simulink model "p1"  (R2021a)
settings: Solver=FixedStepAuto  StartTime=0.0  StopTime=10.0  RelTol=1e-3
settings Model: EnablePacing=on  PacingRate=0.100000  Creator=Abbas  LastModifiedBy=Abbas

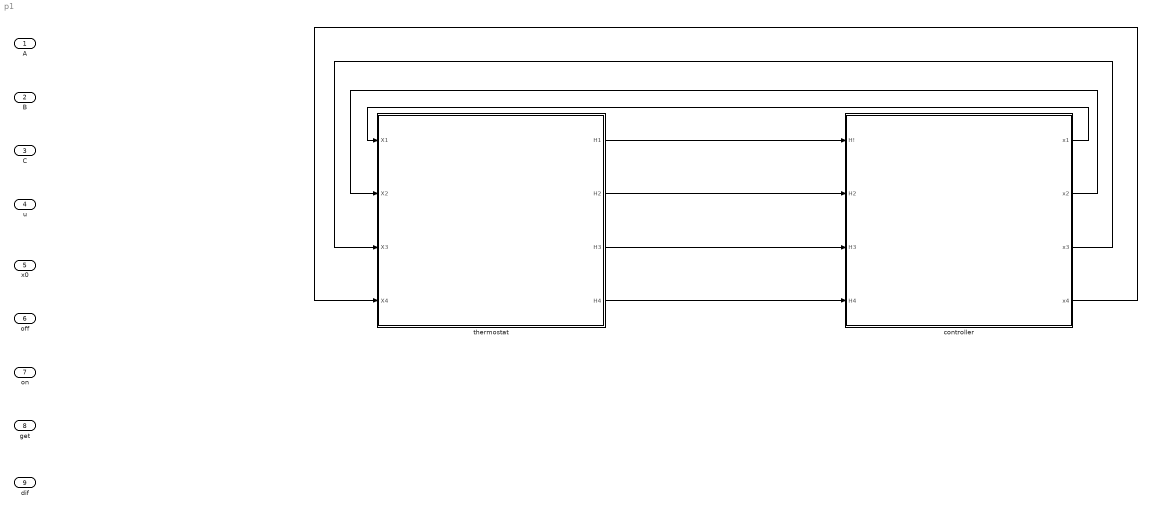
== system p1 ==
  A : Inport
  B : Inport  Port=2
  C : Inport  Port=3
  u : Inport  Port=4
  x0 : Inport  Port=5
  off : Inport  Port=6
  on : Inport  Port=7
  get : Inport  Port=8
  dif : Inport  Port=9
  controller : Subsystem
  thermostat : Subsystem
  wires:
  controller/1(x1) -> thermostat/1(X1)
  thermostat/1(H1) -> controller/1(H!)
  thermostat/2(H2) -> controller/2(H2)
  thermostat/3(H3) -> controller/3(H3)
  thermostat/4(H4) -> controller/4(H4)
  controller/2(x2) -> thermostat/2(X2)
  controller/3(x3) -> thermostat/3(X3)
  controller/4(x4) -> thermostat/4(X4)

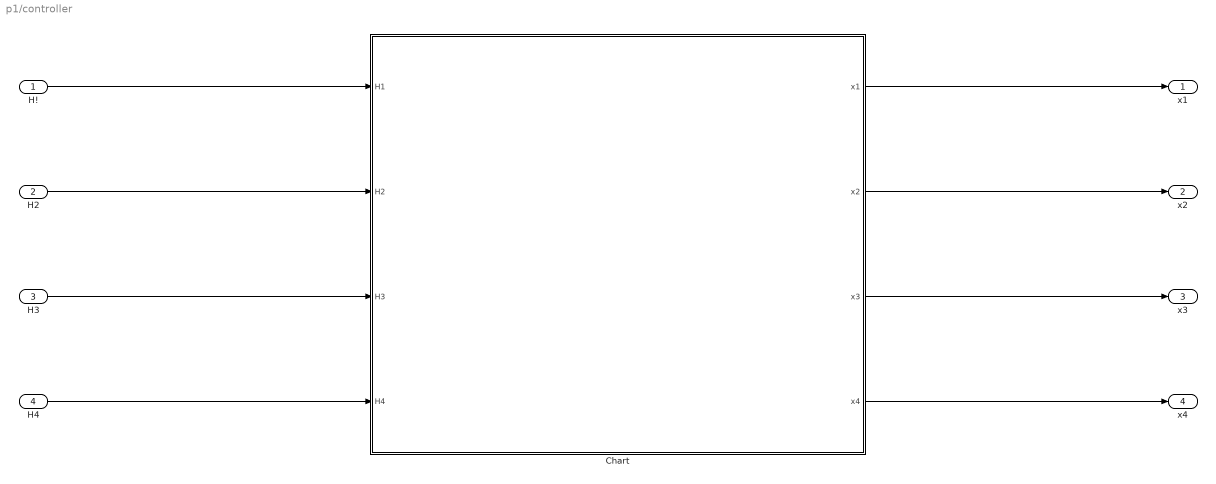
== system p1/controller ==
  H! : Inport
  H2 : Inport  Port=2
  H3 : Inport  Port=3
  H4 : Inport  Port=4
  Chart : Stateflow chart  TreatAsAtomicUnit=on
  x1 : Outport
  x2 : Outport  Port=2
  x3 : Outport  Port=3
  x4 : Outport  Port=4
  wires:
  Chart/1(x1) -> x1/1
  Chart/2(x2) -> x2/1
  Chart/3(x3) -> x3/1
  Chart/4(x4) -> x4/1
  H!/1 -> Chart/1(H1)
  H2/1 -> Chart/2(H2)
  H3/1 -> Chart/3(H3)
  H4/1 -> Chart/4(H4)

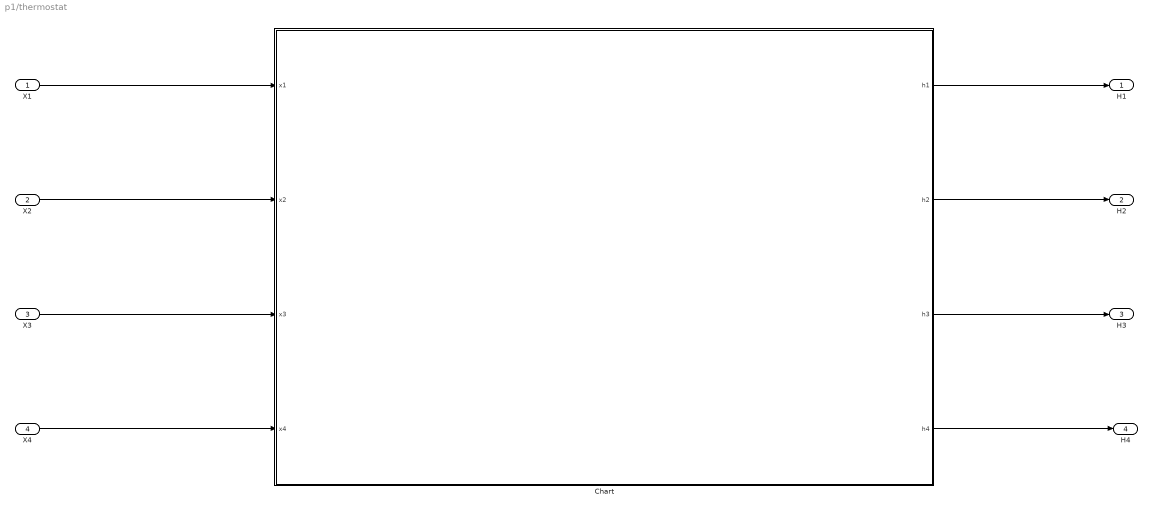
== system p1/thermostat ==
  X1 : Inport
  X2 : Inport  Port=2
  X3 : Inport  Port=3
  X4 : Inport  Port=4
  Chart : Stateflow chart  TreatAsAtomicUnit=on
  H1 : Outport
  H2 : Outport  Port=2
  H3 : Outport  Port=3
  H4 : Outport  Port=4
  wires:
  X2/1 -> Chart/2(x2)
  X1/1 -> Chart/1(x1)
  X3/1 -> Chart/3(x3)
  X4/1 -> Chart/4(x4)
  Chart/1(h1) -> H1/1
  Chart/2(h2) -> H2/1
  Chart/3(h3) -> H3/1
  Chart/4(h4) -> H4/1

== stateflow chart p1/thermostat/Chart ==
  state start
  state s34
    du:
    h1 = 0;
    h2 = 0;
    h3 = 1;
    h4 = 1;
  state s24
    du:
    h1 = 0;
    h2 = 1;
    h3 = 0;
    h4 = 1;
  state s23
    du:
    h1 = 0;
    h2 = 1;
    h3 = 1;
    h4 = 0;
  state snull
    du:
    h1 = 0;
    h2 = 0;
    h3 = 0;
    h4 = 0;
  state s1
    du:
    h1 = 1;
    h2 = 0;
    h3 = 0;
    h4 = 0;
  state s2
    du:
    h1 = 0;
    h2 = 1;
    h3 = 0;
    h4 = 0;
  state s3
    du:
    h1 = 0;
    h2 = 0;
    h3 = 1;
    h4 = 0;
  state s4
    du:
    h1 = 0;
    h2 = 0;
    h3 = 0;
    h4 = 1;
  state s12
    du:
    h1 = 1;
    h2 = 1;
    h3 = 0;
    h4 = 0;
  state s13
    du:
    h1 = 1;
    h2 = 0;
    h3 = 1;
    h4 = 0;
  state s14
    du:
    h1 = 1;
    h2 = 0;
    h3 = 0;
    h4 = 1;
  s14 -> s23 [order 6] : [(x1-x2>=dif2 & x2<=get2 & x4-x3>=dif3 & x3<=get3) | (x4-x2>=dif2 & x2<=get2 & x1-x3>=dif3 & x3<=get3) ]
  s23 -> s14 [order 6] : [(x2-x1>=dif1 & x1<=get1 & x3-x4>=dif4 & x4<=get4) | (x3-x1>=dif1 & x1<=get1 & x2-x4>=dif4 & x4<=get4) ]
  (default) -> start
  start -> s23 : [1==1]
  s14 -> s24 [order 7] : [x1-x2>=dif2 & x2<=get2]
  s24 -> s14 [order 5] : [x2-x1>=dif1 & x1<=get1]
  s24 -> s34 [order 4] : [x2-x3>=dif3 & x3<=get3]
  s23 -> s24 [order 4] : [x3-x4>=dif4 & x4<=get4]
  s34 -> s24 [order 3] : [x3-x2>=dif2 & x2<=get2]
  s14 -> s34 [order 4] : [x1-x3>=dif3 & x3<=get3]
  s34 -> s14 [order 4] : [x3-x1>=dif1 & x1<=get1]
  s13 -> s23 [order 7] : [x1-x2>=dif2 & x2<=get2]
  s3 -> s34 [order 2] : [x4<on4]
  s24 -> s23 [order 3] : [x4-x3>=dif3 & x3<=get3]
  s23 -> s13 [order 7] : [x2-x1>=dif1 & x1<=get1]
  s34 -> s23 [order 5] : [x3-x4>=dif4 & x4<=get4]
  s12 -> s23 [order 3] : [x1-x3>=dif3 & x3<=get3]
  s23 -> s34 [order 1] : [x4-x3>=dif3 & x3<=get3]
  s12 -> s34 [order 5] : [(x1-x3>=dif3 & x3<=get3 & x2-x4>=dif4 & x4<=get4) | (x2-x3>=dif3 & x3<=get3 & x1-x4>=dif4 & x4<=get4)]
  s23 -> s12 [order 5] : [x3-x1>=dif1 & x1<=get1]
  s24 -> s13 [order 6] : [(x2-x3>=dif3 & x3<=get3 & x4-x1>=dif1 & x1<=get1) | (x4-x3>=dif3 & x3<=get3 & x2-x1>=dif1 & x1<=get1)]
  s24 -> s12 [order 7] : [x4-x1>=dif1 & x1<=get1]
  s23 -> s3 [order 2] : [x2>off2]
  s34 -> s12 [order 7] : [(x3-x1>=dif1 & x1<=get1 & x4-x2>=dif2 & x2<=get2) | (x4-x1>=dif1 & x1<=get1 & x3-x2>=dif2 & x2<=get2)]
  s34 -> s3 [order 2] : [x4>off4]
  s13 -> s34 [order 5] : [x1-x4>=dif4 & x4<=get4]
  s34 -> s13 [order 6] : [x4-x1>=dif1 & x1<=get1]
  s4 -> s34 [order 3] : [x3<on3]
  s34 -> s4 [order 1] : [x3>off3]
  s13 -> s24 [order 6] : [(x3-x2>=dif2 & x2<=get2 & x1-x4>=dif4 & x4<=get4) | (x1-x2>=dif2 & x2<=get2 & x3-x4>=dif4 & x4<=get4)]
  s12 -> s24 [order 7] : [x1-x4>=dif4 & x4<=get4]
  s2 -> s23 [order 4] : [x3<on3]
  s24 -> s2 [order 1] : [x4>off4]
  s4 -> s24 [order 4] : [x2<on2]
  s24 -> s4 [order 2] : [x2>off2]
  s23 -> s2 [order 3] : [x3>off3]
  s3 -> s23 [order 3] : [x2<on2]
  s2 -> (junction 203) [order 3] : [x4<on4]
  s1 -> snull [order 1] : [x1>off1]
  s2 -> snull [order 1] : [x2>off2]
  s3 -> snull [order 1] : [x3>off3]
  s4 -> snull [order 1] : [x4>off4]
  s14 -> s1 [order 2] : [x4>off4]
  snull -> s1 [order 1] : [x1<on1]
  s1 -> s12 [order 2] : [x2<on2]
  s12 -> s1 [order 2] : [x2>off2]
  s1 -> s14 [order 4] : [x4<on4]
  s13 -> s1 [order 2] : [x3>off3]
  s1 -> s13 [order 3] : [x3<on3]
  s4 -> s14 [order 2] : [x1<on1]
  snull -> s2 [order 2] : [x2<on2]
  s12 -> s2 [order 1] : [x1>off1]
  s2 -> s12 [order 2] : [x1<on1]
  snull -> s3 [order 3] : [x3<on3]
  s13 -> s3 [order 1] : [x1>off1]
  s3 -> s13 [order 4] : [x1<on1]
  snull -> s4 [order 4] : [x4<on4]
  s14 -> s4 [order 1] : [x1>off1]
  s13 -> s12 [order 4] : [x3-x2>=dif2 & x2<=get2]
  s13 -> s14 [order 3] : [x3-x4>=dif4 & x4<=get4]
  s12 -> s13 [order 4] : [x2-x3>=dif3 & x3<=get3]
  s14 -> s13 [order 5] : [x4-x3>=dif3 & x3<=get3]
  s14 -> s12 [order 3] : [x4-x2>=dif2 & x2<=get2]
  s12 -> s14 [order 6] : [x2-x4>=dif4 & x4<=get4]
  data: on1 local double =19; on2 local double =19; on3 local double =19; on4 local double =19; off1 local double =20; off2 local double =20; off3 local double =20; off4 local double =20; get1 local double =17; get2 local double =16; get3 local double =16; get4 local double =17; dif1 local double =1; dif2 local double =1; dif3 local double =1; dif4 local double =1; x1 input double; x2 input double; x3 input double; x4 input double; h1 output double; h2 output double; h3 output double; h4 output double; x01 local double =16.5; x02 local double =16.5; x03 local double =16.5; x04 local double =16.5

== stateflow chart p1/controller/Chart ==
  settings: updateMethod=CONTINUOUS
  state state_1
    du:
    x1_dot = H1*C1 + B1*(u-x1)+A12*(x1-x2) + A13*(x1-x3) + A14*(x1-x4);
    x2_dot = H2*C2 + B2*(u-x2)+A21*(x2-x1) + A23*(x2-x3) + A24*(x2-x4);
    x3_dot = H3*C3 + B3*(u-x3)+A31*(x3-x1) + A32*(x3-x2) + A34*(x3-x4);
    x4_dot = H4*C4 + B4*(u-x4)+A41*(x4-x1) + A42*(x4-x2) + A43*(x4-x3);
  (default) -> state_1 : {x1 = x01; x2 = x02; x1 = x01; x3 = x03; x4 = x04;}
  data: A12 local =0.3; A13 local =0.4; A14 local =0.3; A21 local =0.3; A23 local =0.5; A24 local =0; A31 local =0.4; A32 local =0.5; A34 local =0.3; A41 local =0.3; A42 local =0; A43 local =0.3; B1 local =0.3; B2 local =0.2; B3 local =0.5; B4 local =0.4; C1 local =9; C2 local =7; C3 local =11; C4 local =7; x01 local =16.5; x02 local =16.5; x03 local =16.5; x04 local =16.5; u local =6; H1 input =0; H2 input =1; H3 input =0; H4 input =1; x1 output; x2 output; x3 output; x4 output
  data x1 settings: updateMethod=SF_CONTINUOUS_TIME_DATA
  data x2 settings: updateMethod=SF_CONTINUOUS_TIME_DATA
  data x3 settings: updateMethod=SF_CONTINUOUS_TIME_DATA
  data x4 settings: updateMethod=SF_CONTINUOUS_TIME_DATA
